simulink subsystem "Make_Knots"  (R2023b)
settings: Solver=VariableStepAuto  StartTime=0.0  StopTime=10.0  RelTol=1e-3
undefined symbols (not defined in the file): Spline_Max_Num_RefPoses, Spline_Velocity_Adjustment_Magnitude
settings Model: Creator=FIRSTMentor  LastModifiedBy=FIRSTMentor

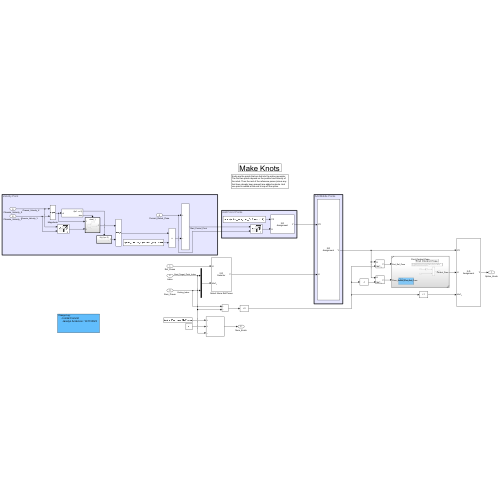
[thumbnail: Simulink's stored preview of the top-level diagram]
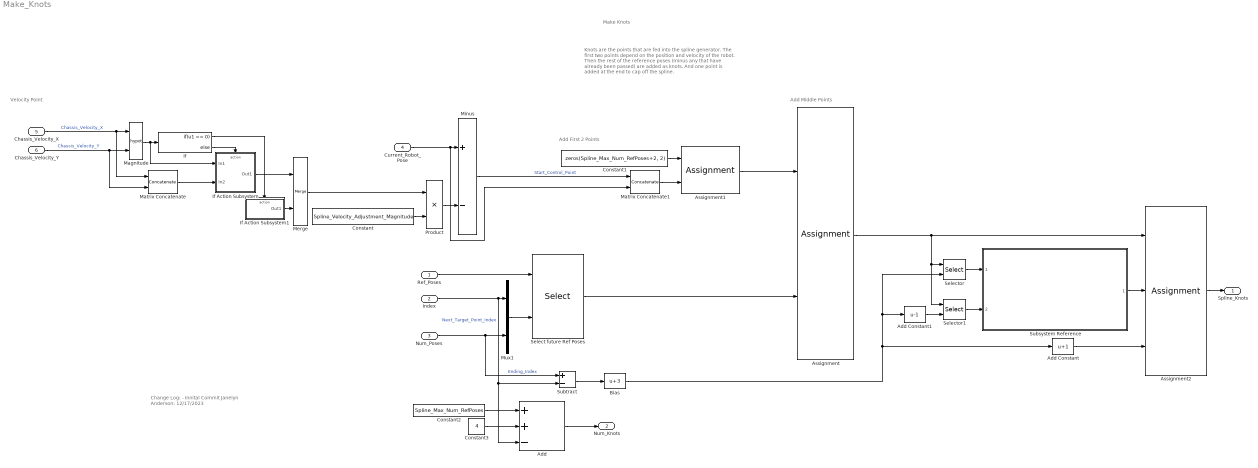
== system Make_Knots ==
  note: Add First 2 Points
  note: Add Middle Points
  note: Velocity Point
  note: Knots are the points that are fed into the spline generator. The first two points depend on the position and velocity of the robot. Then the rest of the reference poses (minus any that have already been passed) are added as knots. And one point is added at the end to cap off the spline.
  note: Make Knots
  note: Change Log:
      | - Innital Commit
      | Janelyn Anderson: 12/17/2023
  Ref_Poses : Inport
  Index : Inport  Port=2
  Num_Poses : Inport  Port=3
  Current_Robot_Pose : Inport  Port=4
  Chassis_Velocity_X : Inport  Port=5
  Chassis_Velocity_Y : Inport  Port=6
  Add : Sum  Inputs=++-
  Add Constant : Bias  Bias=1  SaturateOnIntegerOverflow=off
  Add Constant1 : Bias  Bias=-1  SaturateOnIntegerOverflow=off
  Assignment : Assignment  NumberOfDimensions=2  DiagnosticForDimensions=Warning  IndexOptions=Starting index (dialog),Assign all  Indices=3,1  OutputSizes=1,1
  Assignment1 : Assignment  NumberOfDimensions=2  DiagnosticForDimensions=Warning  IndexOptions=Starting index (dialog),Assign all  Indices=1,1  OutputSizes=1,1
  Assignment2 : Assignment  NumberOfDimensions=2  DiagnosticForDimensions=Warning  IndexOptions=Index vector (port),Assign all  Indices=1,1  OutputSizes=1,1
  Bias : Bias  Bias=3  SaturateOnIntegerOverflow=off
  Constant : Constant  Value=Spline_Velocity_Adjustment_Magnitude
  Constant1 : Constant  Value=zeros(Spline_Max_Num_RefPoses+2, 2)
  Constant2 : Constant  Value=Spline_Max_Num_RefPoses
  Constant3 : Constant  Value=4
  If : If  IfExpression=u1 == 0
  If Action Subsystem : Subsystem  TreatAsAtomicUnit=on
  If Action Subsystem1 : Subsystem  TreatAsAtomicUnit=on
  Magnitude : Math  Operator=hypot
  Matrix Concatenate : Concatenate  Mode=Multidimensional array  ConcatenateDimension=2
  Matrix Concatenate1 : Concatenate  Mode=Multidimensional array
  Merge : Merge
  Minus : Sum  Inputs=+-
  Mux1 : Mux  Inputs=2
  Product : Product
  Select future Ref Poses : Selector  NumberOfDimensions=2  InputPortWidth=3  IndexOptions=Starting and ending indices (port),Select all  Indices=[1 3],1  OutputSizes=1,1
  Selector : Selector  NumberOfDimensions=2  InputPortWidth=3  IndexOptions=Index vector (port),Select all  Indices=[1 3],1  OutputSizes=1,1
  Selector1 : Selector  NumberOfDimensions=2  InputPortWidth=3  IndexOptions=Index vector (port),Select all  Indices=[1 3],1  OutputSizes=1,1
  Subsystem Reference : Subsystem  ReferencedSubsystem=Find_Control_Pose
  Subtract : Sum  Inputs=+-
  Spline_Knots : Outport
  Num_Knots : Outport  Port=2
  wires:
  Bias/1 -> Selector/2, Add Constant1/1, Add Constant/1
  Assignment/1 -> Assignment2/1, Selector/1, Selector1/1
  If/2 -> If Action Subsystem/Action
  Add Constant1/1 -> Selector1/2
  Merge/1 -> Product/1
  Selector1/1 -> Subsystem Reference/2
  If/1 -> If Action Subsystem1/Action
  Assignment2/1 -> Spline_Knots/1
  Ref_Poses/1 -> Select future Ref Poses/1
  Constant/1 -> Product/2
  Select future Ref Poses/1 -> Assignment/2
  If Action Subsystem/1(Out1) -> Merge/1
  Subtract/1 -> Bias/1
  Constant1/1 -> Assignment1/1
  Product/1 -> Minus/2
  Chassis_Velocity_Y/1 -> Matrix Concatenate/2, Magnitude/2  "Chassis_Velocity_Y"
  Constant3/1 -> Add/2
  Selector/1 -> Subsystem Reference/1
  Chassis_Velocity_X/1 -> Matrix Concatenate/1, Magnitude/1  "Chassis_Velocity_X"
  Num_Poses/1 -> Subtract/1, Mux1/2  "Ending_Index"
  Assignment1/1 -> Assignment/1
  Constant2/1 -> Add/1
  Index/1 -> Subtract/2, Add/3, Mux1/1  "Next_Target_Point_Index"
  Matrix Concatenate1/1 -> Assignment1/2
  Add/1 -> Num_Knots/1
  Subsystem Reference/1 -> Assignment2/2
  Add Constant/1 -> Assignment2/3
  Mux1/1 -> Select future Ref Poses/2
  Matrix Concatenate/1 -> If Action Subsystem/2(In2)
  If Action Subsystem1/1(Out1) -> Merge/2
  Minus/1 -> Matrix Concatenate1/1  "Start_Control_Point"
  Magnitude/1 -> If Action Subsystem/1(In1), If/1
  Current_Robot_Pose/1 -> Matrix Concatenate1/2, Minus/1

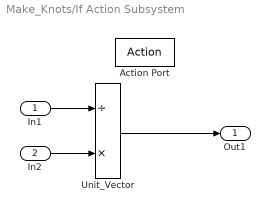
== system Make_Knots/If Action Subsystem ==
  In1 : Inport
  In2 : Inport  Port=2
  Action Port : ActionPort  ActionPortLabel=else
  Unit_Vector : Product  Inputs=/*
  Out1 : Outport
  wires:
  In1/1 -> Unit_Vector/1
  In2/1 -> Unit_Vector/2
  Unit_Vector/1 -> Out1/1

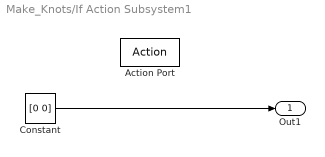
== system Make_Knots/If Action Subsystem1 ==
  Action Port : ActionPort  ActionPortLabel=if(u1 == 0)
  Constant : Constant  Value=[0 0]  VectorParams1D=off
  Out1 : Outport
  wires:
  Constant/1 -> Out1/1
